simulink model "Aug_MPC_CO"  (R2021a)
settings: Solver=FixedStepDiscrete  StartTime=0.0  StopTime=10.0  FixedStep=h  RelTol=1e-3
values from neighbouring files (symbols this model uses):
  A = [0 0 0 0 0 0 0 0 0 -0.534142885228 22.5045950602 -13.9882516442 ... (36 elements, 6x6)]    [Values_Rev3.mat]
  B = [0 0 0 0.425188099574 -0.174236211288 -0.288671680413 0 0 0 -0.174236211288 7.34094843962 -4.56293631615 ... (18 elements, 6x3)]    [Values_Rev3.mat]
  C = sys.C    [Initialize_MPC.m]    (also in Initialize_MPC_non.m; Values_Rev3.mat = [1 0 0 0 1 0 0 0 1 0 0 0 ... (18 elements, 3x6)])
  h = 0.01    [Main_Funwork4.m]
  L = P^-1*Y    [Main_Funwork4.m]    (also in Values_Rev3.mat = [117.002054601 0.873440159496 -0.454542417964 4786.49521284 )
  m = 3    [Main_Funwork4.m]
  Np = 43    [Main_Funwork4.m]
  r_p = zeros(m*Np,1)    [Initialize_MPC.m]    (also in Initialize_MPC_non.m = zeros(3*Np,1))
  u_e = [0 9.21172186389 3.90190360694]    [Values_Rev3.mat]
  x_e = [0.1 -1.0471975512 -0.785398163397 0 0 0]    [Values_Rev3.mat]
undefined symbols (not defined in the file or in its folder): constraints, DiscIntNeverNeededParam, int, matrices, x0
libraries: vrlib x2, simulink x1, aerolibanimutils x1, dspvision x1
settings Model: Creator=vicen  LastModifiedBy=vicen

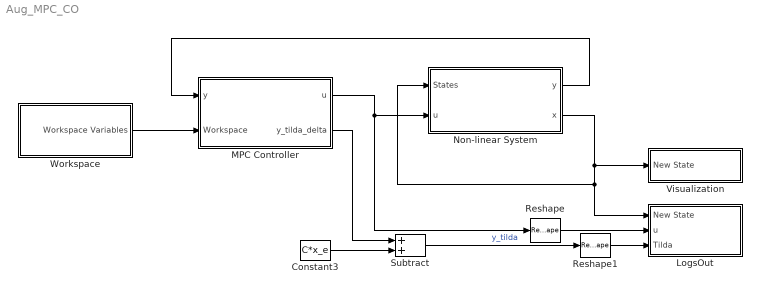
== system Aug_MPC_CO ==
  Constant3 : Constant  Value=C*x_e
  LogsOut : Subsystem
  MPC Controller : Subsystem
  Non-linear System : Subsystem
  Reshape : Reshape
  Reshape1 : Reshape
  Subtract : Sum
  Visualization : Subsystem
  Workspace : Subsystem
  wires:
  MPC Controller/1(u) -> Reshape/1, Non-linear System/2(u)
  Non-linear System/1(y) -> MPC Controller/1(y)
  Workspace/1(Workspace Variables) -> MPC Controller/2(Workspace)
  Non-linear System/2(x) -> Visualization/1(New State), LogsOut/1(New State), Non-linear System/1(States)
  Reshape/1 -> LogsOut/2(u)
  MPC Controller/2(y_tilda_delta) -> Subtract/1
  Reshape1/1 -> LogsOut/3(Tilda)
  Subtract/1 -> Reshape1/1  "y_tilda"
  Constant3/1 -> Subtract/2

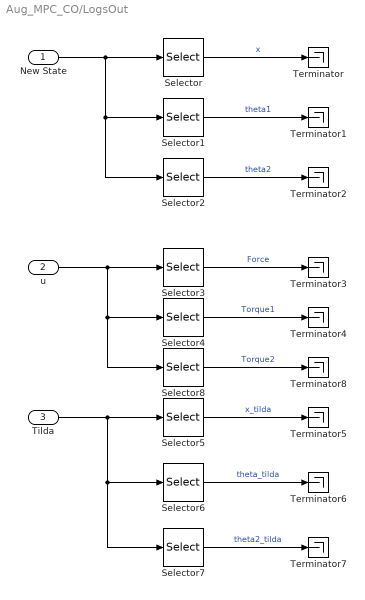
== system Aug_MPC_CO/LogsOut ==
  New State : Inport
  u : Inport  Port=2
  Tilda : Inport  Port=3
  Selector : Selector  InputPortWidth=6  IndexOptions=Index vector (dialog)  Indices=1  OutputSizes=1
  Selector1 : Selector  InputPortWidth=6  IndexOptions=Index vector (dialog)  Indices=2  OutputSizes=1
  Selector2 : Selector  InputPortWidth=6  IndexOptions=Index vector (dialog)  Indices=3  OutputSizes=1
  Selector3 : Selector  InputPortWidth=3  IndexOptions=Index vector (dialog)  Indices=1  OutputSizes=1
  Selector4 : Selector  InputPortWidth=3  IndexOptions=Index vector (dialog)  Indices=2  OutputSizes=1
  Selector5 : Selector  InputPortWidth=3  IndexOptions=Index vector (dialog)  Indices=1  OutputSizes=1
  Selector6 : Selector  InputPortWidth=3  IndexOptions=Index vector (dialog)  Indices=2  OutputSizes=1
  Selector7 : Selector  InputPortWidth=3  IndexOptions=Index vector (dialog)  Indices=3  OutputSizes=1
  Selector8 : Selector  InputPortWidth=3  IndexOptions=Index vector (dialog)  Indices=3  OutputSizes=1
  Terminator{,1..8} (9 alike) : Terminator
  wires:
  Selector/1 -> Terminator/1  "x"
  Selector1/1 -> Terminator1/1  "theta1"
  Selector2/1 -> Terminator2/1  "theta2"
  New State/1 -> Selector2/1, Selector1/1, Selector/1
  u/1 -> Selector8/1, Selector4/1, Selector3/1
  Selector4/1 -> Terminator4/1  "Torque1"
  Selector3/1 -> Terminator3/1  "Force"
  Selector5/1 -> Terminator5/1  "x_tilda"
  Selector6/1 -> Terminator6/1  "theta_tilda"
  Selector7/1 -> Terminator7/1  "theta2_tilda"
  Selector8/1 -> Terminator8/1  "Torque2"
  Tilda/1 -> Selector7/1, Selector6/1, Selector5/1

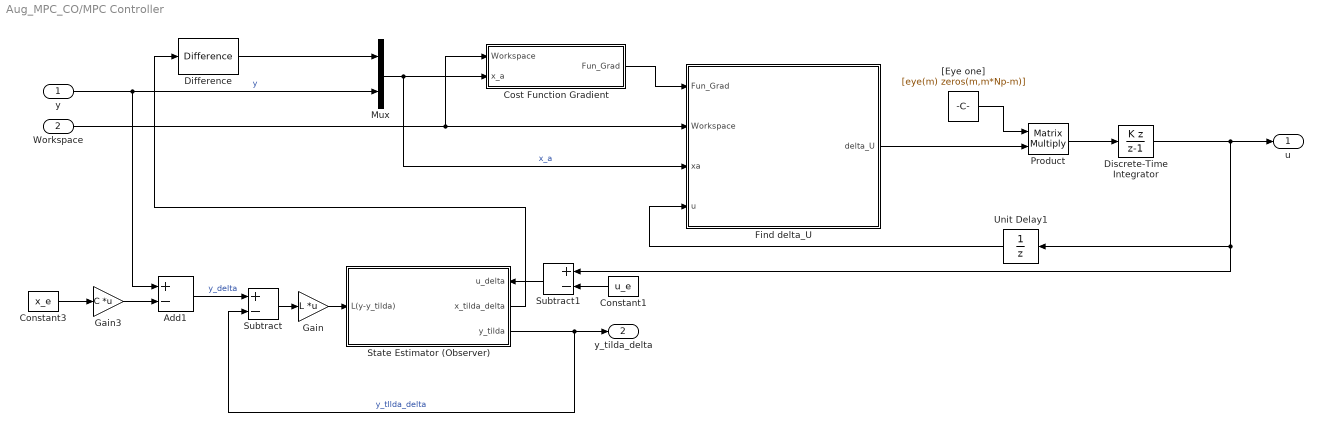
== system Aug_MPC_CO/MPC Controller ==
  y : Inport
  Workspace : Inport  Port=2
  Add1 : Sum  Inputs=+-
  Constant1 : Constant  Value=u_e
  Constant3 : Constant  Value=x_e
  Cost Function Gradient : Subsystem
  Difference : simulink/Discrete/Difference  ICPrevInput=[x0.x;x0.theta1;x0.theta2;x0.x_dot;x0.theta1_dot;x0.theta2_dot]  OutMin=[]  OutMax=[]  OutDataType=fixdt(1, 16)  OutScaling=2^-10  DoSatur=off
  Discrete-Time Integrator : DiscreteIntegrator  IntegratorMethod=Accumulation: Backward Euler  InitialCondition=[0;0;0]  SampleTime=-1  ICPrevOutput=DiscIntNeverNeededParam  ICPrevScaledInput=DiscIntNeverNeededParam
  Find delta_U : Subsystem
  Gain : Gain  Gain=L  Multiplication=Matrix(K*u)
  Gain3 : Gain  Gain=C  Multiplication=Matrix(K*u)
  Mux : Mux  Inputs=2
  Product : Product  Multiplication=Matrix(*)  OutDataTypeStr=Inherit: Inherit via back propagation
  State Estimator (Observer) : Subsystem
      settings: PortSchema="{\"entries\":[{\"content\":{\"sides\":[{\"content\":{\"connectorIds\":[\"In1\"]},\"type\":\"ConnectorPlacement.EquallySpacedRectSide\",\"uuid\":\"57453572-00db-41c9-97df-639cc5f0b98d\"},{\"content\":{\"connectorIds\":[\"In2\",\"Out1\",\"Out2\"],\"side\":\"RIGHT\"},\"type\":\"ConnectorPlacement.EquallySpacedRectSide\",\"uuid\":\"3b8eab05-1f6d-4087-8816-503eb36a27cc\"},{\"content\":{\"connectorIds\":[],\"side\":\"TOP\"},\"type\":\"ConnectorPlacement.EquallySpacedRectSide\",\"uuid\":\"5deb75af-e21c-47dc-bc74-f1da50ac49fd\"}]},\"type\":\"ConnectorPlacement.EquallySpacedConnector\",\"uuid\":\"2f660e10-f165-4d4d-b1be-120147264fde\"}],\"packageUris\":[\"http://schema.mathworks.com/mf0/Connector/R2020b\"],\"version\":\"1.0\"}"
  Subtract : Sum  Inputs=+-
  Subtract1 : Sum  Inputs=+-
  Unit Delay1 : UnitDelay  InitialCondition=[0;0;0]  SampleTime=-1  HasFrameUpgradeWarning=on
  "[Eye one]" : Constant  Value=[eye(m) zeros(m,m*Np-m)]  VectorParams1D=off
  u : Outport
  y_tilda_delta : Outport  Port=2
  wires:
  Difference/1 -> Mux/1
  "[Eye one]"/1 -> Product/1
  Workspace/1 -> Find delta_U/2(Workspace), Cost Function Gradient/1(Workspace)
  Mux/1 -> Cost Function Gradient/2(x_a), Find delta_U/3(xa)  "x_a"
  Find delta_U/1(delta_U) -> Product/2
  Cost Function Gradient/1(Fun_Grad) -> Find delta_U/1(Fun_Grad)
  Product/1 -> Discrete-Time Integrator/1
  Discrete-Time Integrator/1 -> Subtract1/1, Unit Delay1/1, u/1
  Unit Delay1/1 -> Find delta_U/4(u)
  Add1/1 -> Subtract/1  "y_delta"
  y/1 -> Add1/1, Mux/2  "y"
  Constant3/1 -> Gain3/1
  Subtract/1 -> Gain/1
  Gain/1 -> State Estimator (Observer)/1(L(y-y_tilda))
  Gain3/1 -> Add1/2
  State Estimator (Observer)/2(y_tilda) -> Subtract/2, y_tilda_delta/1  "y_tllda_delta"
  Constant1/1 -> Subtract1/2
  Subtract1/1 -> State Estimator (Observer)/2(u_delta)
  State Estimator (Observer)/1(x_tilda_delta) -> Difference/1

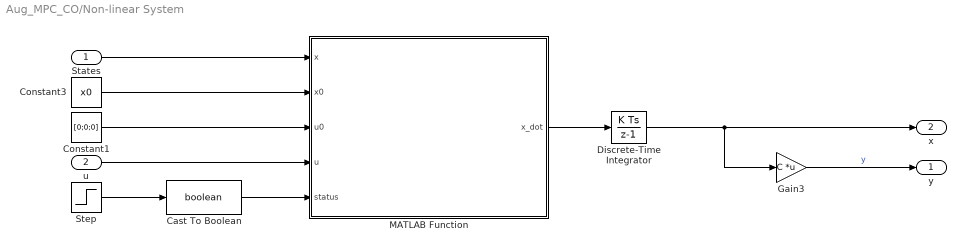
== system Aug_MPC_CO/Non-linear System ==
  States : Inport
  u : Inport  Port=2
  Cast To Boolean : DataTypeConversion  OutDataTypeStr=boolean
  Constant1 : Constant  Value=[0;0;0]  VectorParams1D=off
  Constant3 : Constant  Value=x0  VectorParams1D=off  OutDataTypeStr=Bus: State_bus
  Discrete-Time Integrator : DiscreteIntegrator  InitialCondition=[x0.x;x0.theta1;x0.theta2;x0.x_dot;x0.theta1_dot;x0.theta2_dot]  SampleTime=h  ICPrevOutput=DiscIntNeverNeededParam  ICPrevScaledInput=DiscIntNeverNeededParam
  Gain3 : Gain  Gain=C  Multiplication=Matrix(K*u)
  MATLAB Function : MATLAB Function  TreatAsAtomicUnit=on
  Step : Step  Time=h  SampleTime=0
  y : Outport
  x : Outport  Port=2
  wires:
  States/1 -> MATLAB Function/1(x)
  u/1 -> MATLAB Function/4(u)
  Step/1 -> Cast To Boolean/1
  Cast To Boolean/1 -> MATLAB Function/5(status)
  Gain3/1 -> y/1  "y"
  Constant3/1 -> MATLAB Function/2(x0)
  MATLAB Function/1(x_dot) -> Discrete-Time Integrator/1
  Constant1/1 -> MATLAB Function/3(u0)
  Discrete-Time Integrator/1 -> Gain3/1, x/1

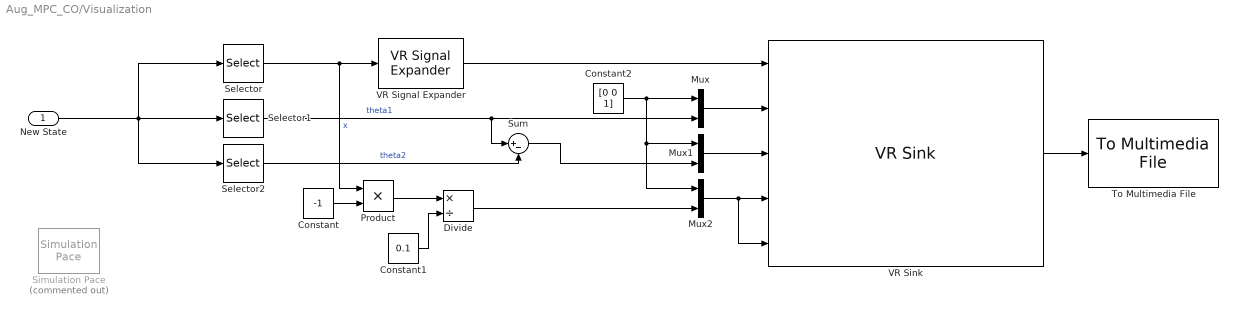
== system Aug_MPC_CO/Visualization ==
  New State : Inport
  Constant : Constant  Value=-1
  Constant1 : Constant  Value=0.1
  Constant2 : Constant  Value=[0 0 1]
  Divide : Product  Inputs=*/
  Mux : Mux  Inputs=2
  Mux1 : Mux  Inputs=2
  Mux2 : Mux  Inputs=2
  Product : Product
  Selector : Selector  InputPortWidth=6  IndexOptions=Index vector (dialog)  Indices=1  OutputSizes=1
  Selector1 : Selector  InputPortWidth=6  IndexOptions=Index vector (dialog)  Indices=2  OutputSizes=1
  Selector2 : Selector  InputPortWidth=6  IndexOptions=Index vector (dialog)  Indices=3  OutputSizes=1
  Simulation Pace : aerolibanimutils/Simulation Pace  Commented=on  SimulationPace=1  SleepMode=Auto  OutputPaceError=off  SampleTime=1/30
  Sum : Sum  Inputs=|+-
  To Multimedia File : dspvision/To Multimedia File  outputFilename=test.avi  streamSelection=Video only  videoCompressor=None (uncompressed)  audioCompressor=None (uncompressed)  imagePorts=One multidimensional signal  fileType=AVI  audioDatatype=Determine from input data type  fourcc=RGB  videoQuality=75  mj2000CompFactor=10
  VR Signal Expander : vrlib/VR Signal Expander  outwidth=3  outidx=[1]
  VR Sink : vrlib/VR Sink  InstantiateOnLoad=on  SampleTime=0.1  ViewEnable=on  RemoteChange=off  RemoteView=off  FieldsWritten=Cart.translation.3.1.1.double#Rotation1.rotation.4.1.1.double#Rotation2.rotation.4.1.1.double#Axis_Rotate.rotation.4.1.1.double#Axis_Rotate2.rotation.4.1.1.double  WorldFileName=Cart_Actual.WRL  AutoView=off  VideoDimensions=[1500 2000]  AllowVariableSize=off  FigureProperties="{'Position', 'Name', 'Viewpoint', 'CameraBound', 'CameraDirection', 'CameraPosition', 'CameraUpVector', 'ZoomFactor', 'Antialiasing', 'Headlight', 'Lighting', 'NavPanel', 'Sound', 'StatusBar', 'Stereo3D', 'Stereo3DCameraOffset', 'Stereo3DHIT', 'ToolBar', 'Textures', 'Transparency', 'Triad', 'Wireframe', 'NavZones', 'NavMode', 'NavSpeed', 'CaptureFileFormat', 'CaptureFileName', 'Record2DCompressMethod', 'Record2DCompressQuality', 'Record2D', 'Record2DFileName', 'Record2DFPS'; [1.2660000000000001e+02   9.4799999999999955e+01   8.0000000000000000e+02   6.0020000000000005e+02], '', '_untitled_1', 'on', [0.0000000000000000e+00   0.0000000000000000e+00  -1.0000000000000000e+00], [0.0000000000000000e+00   0.0000000000000000e+00   0.0000000000000000e+00], [0.0000000000000000e+00   1.0000000000000000e+00   0.0000000000000000e+00], [1.0000000000000000e+00], 'on', 'on', 'on', 'none', 'on', 'off', 'off', [1.0000000149011612e-01], [0.0000000000000000e+00], 'off', 'on', 'on', 'none', 'off', 'off', 'fly', 'normal', 'tif', '%f_anim_%n.tif', 'auto', [7.5000000000000000e+01], 'off', '***video***', 'auto'}"
  wires:
  New State/1 -> Selector/1, Selector2/1, Selector1/1
  Selector/1 -> VR Signal Expander/1, Product/1  "x"
  Selector1/1 -> Sum/1, Mux/2  "theta1"
  Product/1 -> Divide/1
  Constant/1 -> Product/2
  Constant1/1 -> Divide/2
  Constant2/1 -> Mux1/1, Mux2/1, Mux/1
  Selector2/1 -> Sum/2  "theta2"
  Divide/1 -> Mux2/2
  Sum/1 -> Mux1/2
  VR Signal Expander/1 -> VR Sink/1
  Mux/1 -> VR Sink/2
  Mux1/1 -> VR Sink/3
  Mux2/1 -> VR Sink/4, VR Sink/5
  VR Sink/1 -> To Multimedia File/1

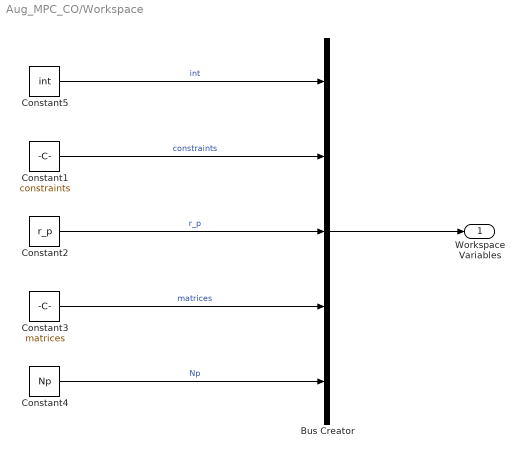
== system Aug_MPC_CO/Workspace ==
  Bus Creator : BusCreator  Inputs=5
  Constant1 : Constant  Value=constraints  VectorParams1D=off  OutDataTypeStr=Bus: Contraint_bus
  Constant2 : Constant  Value=r_p
  Constant3 : Constant  Value=matrices  VectorParams1D=off  OutDataTypeStr=Bus: Matrix_bus
  Constant4 : Constant  Value=Np  VectorParams1D=off
  Constant5 : Constant  Value=int  VectorParams1D=off  OutDataTypeStr=Bus: Initial_bus
  Workspace Variables : Outport
  wires:
  Bus Creator/1 -> Workspace Variables/1
  Constant1/1 -> Bus Creator/2  "constraints"
  Constant2/1 -> Bus Creator/3  "r_p"
  Constant3/1 -> Bus Creator/4  "matrices"
  Constant4/1 -> Bus Creator/5  "Np"
  Constant5/1 -> Bus Creator/1  "int"

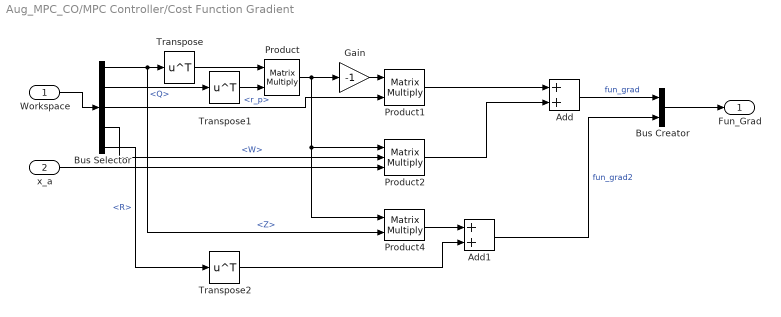
== system Aug_MPC_CO/MPC Controller/Cost Function Gradient ==
  Workspace : Inport
  x_a : Inport  Port=2
  Add : Sum
  Add1 : Sum
  Bus Creator : BusCreator  Inputs=2
  Bus Selector : BusSelector  OutputSignals=matrices.Z,matrices.Q,r_p,matrices.W,matrices.R
  Gain : Gain  Gain=-1
  Product : Product  Multiplication=Matrix(*)
  Product1 : Product  Multiplication=Matrix(*)
  Product2 : Product  Inputs=3  Multiplication=Matrix(*)
  Product4 : Product  Multiplication=Matrix(*)
  Transpose : Math  Operator=transpose  SaturateOnIntegerOverflow=on
  Transpose1 : Math  Operator=transpose  SaturateOnIntegerOverflow=on
  Transpose2 : Math  Operator=transpose  SaturateOnIntegerOverflow=on
  Fun_Grad : Outport
  wires:
  Bus Creator/1 -> Fun_Grad/1
  Workspace/1 -> Bus Selector/1
  Bus Selector/1 -> Product4/2, Transpose/1  "<Z>"
  Bus Selector/2 -> Transpose1/1  "<Q>"
  Transpose1/1 -> Product/2
  Product/1 -> Product4/1, Product2/1, Gain/1
  Transpose/1 -> Product/1
  Gain/1 -> Product1/1
  x_a/1 -> Product2/3
  Product1/1 -> Add/1
  Product2/1 -> Add/2
  Add/1 -> Bus Creator/1  "fun_grad"
  Product4/1 -> Add1/1
  Transpose2/1 -> Add1/2
  Add1/1 -> Bus Creator/2  "fun_grad2"
  Bus Selector/4 -> Product2/2  "<W>"
  Bus Selector/5 -> Transpose2/1  "<R>"
  Bus Selector/3 -> Product1/2  "<r_p>"

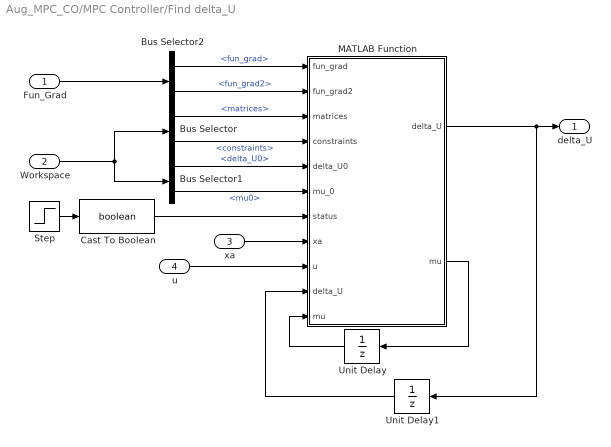
== system Aug_MPC_CO/MPC Controller/Find delta_U ==
  Fun_Grad : Inport
  Workspace : Inport  Port=2
  xa : Inport  Port=3
  u : Inport  Port=4
  Bus Selector : BusSelector  OutputSignals=matrices,constraints
  Bus Selector1 : BusSelector  OutputSignals=int.delta_U0,int.mu0
  Bus Selector2 : BusSelector  OutputSignals=fun_grad,fun_grad2
  Cast To Boolean : DataTypeConversion  OutDataTypeStr=boolean
  MATLAB Function : MATLAB Function  TreatAsAtomicUnit=on
  Step : Step  Time=h-0.001  SampleTime=0
  Unit Delay : UnitDelay  InitialCondition=int.mu0  SampleTime=-1  HasFrameUpgradeWarning=on
  Unit Delay1 : UnitDelay  InitialCondition=int.delta_U0  SampleTime=-1  HasFrameUpgradeWarning=on
  delta_U : Outport
  wires:
  Workspace/1 -> Bus Selector1/1, Bus Selector/1
  Bus Selector/1 -> MATLAB Function/3(matrices)  "<matrices>"
  Bus Selector/2 -> MATLAB Function/4(constraints)  "<constraints>"
  Bus Selector1/2 -> MATLAB Function/6(mu_0)  "<mu0>"
  Bus Selector1/1 -> MATLAB Function/5(delta_U0)  "<delta_U0>"
  Cast To Boolean/1 -> MATLAB Function/7(status)
  Step/1 -> Cast To Boolean/1
  Bus Selector2/1 -> MATLAB Function/1(fun_grad)  "<fun_grad>"
  Bus Selector2/2 -> MATLAB Function/2(fun_grad2)  "<fun_grad2>"
  Fun_Grad/1 -> Bus Selector2/1
  xa/1 -> MATLAB Function/8(xa)
  u/1 -> MATLAB Function/9(u)
  MATLAB Function/2(mu) -> Unit Delay/1
  MATLAB Function/1(delta_U) -> Unit Delay1/1, delta_U/1
  Unit Delay1/1 -> MATLAB Function/10("delta_U ")
  Unit Delay/1 -> MATLAB Function/11("mu ")

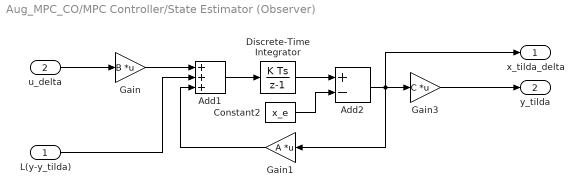
== system Aug_MPC_CO/MPC Controller/State Estimator (Observer) ==
  L(y-y_tilda) : Inport
  u_delta : Inport  Port=2
  Add1 : Sum  Inputs=+++
  Add2 : Sum  Inputs=+-
  Constant2 : Constant  Value=x_e
  Discrete-Time Integrator : DiscreteIntegrator  InitialCondition=[x0.x;x0.theta1;x0.theta2;x0.x_dot;x0.theta1_dot;x0.theta2_dot]  SampleTime=h  ICPrevOutput=DiscIntNeverNeededParam  ICPrevScaledInput=DiscIntNeverNeededParam
  Gain : Gain  Gain=B  Multiplication=Matrix(K*u)
  Gain1 : Gain  Gain=A  Multiplication=Matrix(K*u)
  Gain3 : Gain  Gain=C  Multiplication=Matrix(K*u)
  x_tilda_delta : Outport
  y_tilda : Outport  Port=2
  wires:
  Gain1/1 -> Add1/3
  Add1/1 -> Discrete-Time Integrator/1
  Gain/1 -> Add1/1
  u_delta/1 -> Gain/1
  Gain3/1 -> y_tilda/1
  L(y-y_tilda)/1 -> Add1/2
  Constant2/1 -> Add2/2
  Add2/1 -> Gain3/1, Gain1/1, x_tilda_delta/1
  Discrete-Time Integrator/1 -> Add2/1

== matlab function Aug_MPC_CO/MPC Controller/Find delta_U/MATLAB Function ==
  data: fun_grad input; delta_U output; fun_grad2 input; matrices input; constraints input; delta_U0 input; mu_0 input; status input; xa input; u input; delta_U input size=[69,1]; mu input size=[276,1]; mu output
function [delta_U,mu] = for_loop(fun_grad,fun_grad2,matrices,constraints,delta_U0,mu_0,status,xa,u,delta_U,mu)
    
    % Set-Up
    Dg = [matrices.Z_aug;matrices.H_aug];
    temp = [-constraints.Y_min + matrices.W*xa;
            constraints.Y_max - matrices.W*xa;
           -constraints.U_min + matrices.E*u;
            constraints.U_max - matrices.E*u];
    alpha = 0.01;
    beta = 0.01;
    
    % Check if initial value
    if status == true
        % Do nothing
    else
        delta_U = delta_U0;
        mu = mu_0;
    end
    
    % Find new delta_U
    for i = 1:1000
        gf = fun_grad + fun_grad2*delta_U;
        g_con = Dg*delta_U - temp;
        
        % cnts1 also happens to be the gradient of contraints
        next_delta_U = delta_U - alpha*(gf+Dg'*mu);
        mu = max(mu + beta*g_con,0);        
        
        if abs(next_delta_U - delta_U) < 1.0e-5
           break; 
        end
        delta_U = next_delta_U;
    end
    
    % Check if initial value
    if status == true
        % Do nothing
    else
        delta_U = delta_U0;
        mu = mu_0;
    end
end

== matlab function Aug_MPC_CO/Non-linear System/MATLAB Function ==
  data: x input; x0 input; u0 input; u input; x_dot output; status input
function x_dot  = Nonlinear_Dynamics(x,x0,u0,u,status)
    if status == false
        x2 = x0.theta1;
        x3 = x0.theta2;
        x4 = x0.x_dot;
        x5 = x0.theta1_dot;
        x6 = x0.theta2_dot;
        u1 = u0(1);
        u2 = u0(2);
        u3 = u0(3);
    else
        x2 = x(2);
        x3 = x(3);
        x4 = x(4);
        x5 = x(5);
        x6 = x(6);
        u1 = u(1);
        u2 = u(2);
        u3 = u(3);
    end
    % Insert Equations
    x_dot = double([
                     x4;
                     x5;
                     x6;
                     -(420*u1 - (2943*sin(2*x2))/2 + 150*x5^2*sin(x2) + (135*x6^2*sin(x3))/2 - 180*u1*cos(2*x2 - 2*x3) + 400*u3*cos(2*x2 - x3) - 840*u2*cos(x2) + 840*u3*cos(x2) - 400*u3*cos(x3) + (135*x6^2*sin(2*x2 - x3))/2 + 360*u2*cos(x2 - 2*x3) - 360*u3*cos(x2 - 2*x3))/(30*(5*cos(2*x2) + 9*cos(2*x2 - 2*x3) - 26));
                     (22800*u3 - 22800*u2 - 26487*sin(x2 - 2*x3) - 91233*sin(x2) + 3600*u2*cos(2*x3) - 3600*u3*cos(2*x3) + 4725*x6^2*sin(x2 - x3) + 750*x5^2*sin(2*x2) - 4000*u3*cos(x2 + x3) + 4200*u1*cos(x2) + 1350*x5^2*sin(2*x2 - 2*x3) - 1800*u1*cos(x2 - 2*x3) + 13600*u3*cos(x2 - x3) + 675*x6^2*sin(x2 + x3))/(150*(5*cos(2*x2) + 9*cos(2*x2 - 2*x3) - 26));
                     -(2700*sin(x2 - x3)*x5^2 + 1215*sin(2*x2 - 2*x3)*x6^2 + 13600*u3 - 26487*sin(2*x2 - x3) + 26487*sin(x3) - 4000*u3*cos(2*x2) + 1800*u1*cos(2*x2 - x3) + 3600*u2*cos(x2 + x3) - 3600*u3*cos(x2 + x3) - 1800*u1*cos(x3) - 12240*u2*cos(x2 - x3) + 12240*u3*cos(x2 - x3))/(135*(5*cos(2*x2) + 9*cos(2*x2 - 2*x3) - 26))
                ]);
            
end
